simulink model "cascade-controller-design_1_sim"  (R2023b)
settings: Solver=VariableStepAuto  StartTime=0.0  StopTime=10.0  RelTol=1e-3
values from neighbouring files (symbols this model uses):
  C_d = c2d(C, T_s, 'tustin')    [cascade-controller-design_1.m]    (also in cascade_controller_design_1.m; cascade_controller_design_2.m = c2d(C, T_s, 'zoh'))
  delta_y = 0    [cascade-controller-design_1.m]    (also in cascade_controller_design_1.m; cascade_controller_design_2.m)
  G = 2 / ( (1 + 0.2 * s) * (1 + 0.1 * s) )    [cascade-controller-design_1.m]    (also in cascade_controller_design_1.m; cascade_controller_design_2.m = 0.5 / (s * (1 + s)))
  slope = 0    [cascade-controller-design_1.m]    (also in cascade_controller_design_1.m; cascade_controller_design_2.m)
  step_value = 1    [cascade-controller-design_1.m]    (also in cascade_controller_design_1.m; cascade_controller_design_2.m)
  T_s = 0.001    [cascade-controller-design_1.m]    (also in cascade_controller_design_1.m; cascade_controller_design_2.m)
libraries: cstblocks x2, simulink x1
settings Model: Creator=Atabay  LastModifiedBy=Atabay

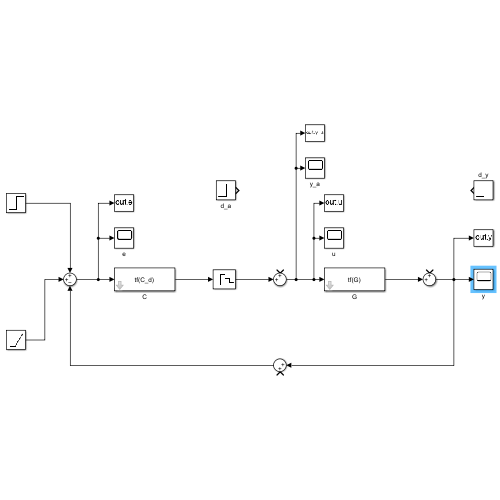
[thumbnail: Simulink's stored preview of the top-level diagram]
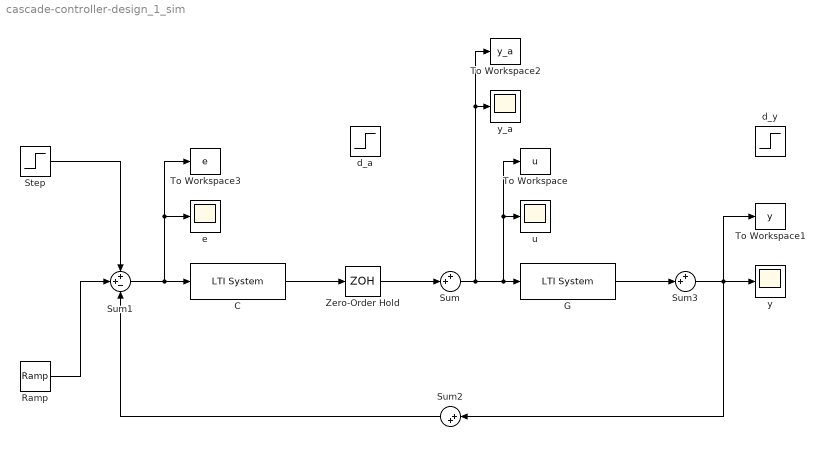
== system cascade-controller-design_1_sim ==
  C : cstblocks/LTI System  sys=tf(C_d)  IC=[]  PadeOrder=0
  G : cstblocks/LTI System  sys=tf(G)  IC=[]  PadeOrder=0
  Ramp : simulink/Sources/Ramp  slope=slope  start=0  InitialOutput=0
  Step : Step  After=step_value  SampleTime=T_s
  Sum : Sum  Inputs=++|
  Sum1 : Sum  Inputs=++-
  Sum2 : Sum  Inputs=|++
  Sum3 : Sum  Inputs=++|
  To Workspace : ToWorkspace  VariableName=u  SaveFormat=Timeseries  SampleTime=-1
  To Workspace1 : ToWorkspace  VariableName=y  SaveFormat=Timeseries  SampleTime=-1
  To Workspace2 : ToWorkspace  VariableName=y_a  SaveFormat=Timeseries  SampleTime=-1
  To Workspace3 : ToWorkspace  VariableName=e  SaveFormat=Timeseries  SampleTime=-1
  Zero-Order Hold : ZeroOrderHold  SampleTime=-1
  d_a : Step  SampleTime=0
  d_y : Step  Time=delta_y  SampleTime=0
  e : Scope
  u : Scope
  y : Scope
  y_a : Scope
  wires:
  G/1 -> Sum3/2
  Sum/1 -> y_a/1, To Workspace2/1, To Workspace/1, u/1, G/1
  C/1 -> Zero-Order Hold/1
  Sum3/1 -> To Workspace1/1, Sum2/1, y/1
  Sum1/1 -> To Workspace3/1, e/1, C/1
  Zero-Order Hold/1 -> Sum/2
  Sum2/1 -> Sum1/3
  Ramp/1 -> Sum1/2
  Step/1 -> Sum1/1
